simulink model "vehicle_14dof_complete"  (R2025a)
settings: Solver=ode23s  StartTime=0.0  StopTime=10  MaxStep=0.01  RelTol=1e-4  AbsTol=1e-5
model workspace (MAT data in the model file):
  ARB_CONFIG = 2
  MANEUVER_TYPE = 1
  params.vehicle.m = 1905
  params.vehicle.m_s = 1525
  params.vehicle.m_u = 95.5
  params.vehicle.I_xx = 734.04
  params.vehicle.I_yy = 2600
  params.vehicle.I_zz = 2900
  params.vehicle.I_xz = 0
  params.vehicle.I_w = 1
  params.vehicle.a = 1.216
  params.vehicle.b = 1.502
  params.vehicle.L = 2.718
  params.vehicle.w = 1.405
  params.vehicle.t_f = 0.7025
  params.vehicle.t_r = 0.7025
  params.vehicle.hu_cg = 0.5
  params.vehicle.hr_cg = 0.5
  params.vehicle.h_cgM = 0.6629
  params.vehicle.R_w = 0.329
  params.vehicle.k_sf = 75000
  params.vehicle.k_sr = 70000
  params.vehicle.c_sf = 5000
  params.vehicle.c_sr = 4000
  params.vehicle.k_t = 200000
  params.vehicle.L_arb_f = 0.5
  params.vehicle.L_arb_r = 0.5
  params.vehicle.k_arb_f = 12.217304764
  params.vehicle.k_arb_r = 6.98131700798
  params.vehicle.pid_f.Kp = 23.15
  params.vehicle.pid_f.Ki = 10.2
  params.vehicle.pid_f.Kd = 5.4
  params.vehicle.pid_r.Kp = 23.15
  params.vehicle.pid_r.Ki = 10.2
  params.vehicle.pid_r.Kd = 5.4
  params.vehicle.T_aarb_max = 0
  params.vehicle.steering_ratio = 18.5
  params.vehicle.delta_max = 0.698131700798
  params.vehicle.arb_active = 0
  params.tire.mu = 1
  params.tire.mu_r = 0.015
  params.tire.pacejka.fy.a1 = -22.1
  params.tire.pacejka.fy.a2 = 1011
  params.tire.pacejka.fy.a3 = 1078
  params.tire.pacejka.fy.a4 = 1.82
  params.tire.pacejka.fy.a5 = 0.208
  params.tire.pacejka.fy.a6 = 0
  params.tire.pacejka.fy.a7 = -0.354
  params.tire.pacejka.fy.a8 = 0.707
  params.tire.pacejka.fy.C = 1.3
  params.tire.pacejka.fx.a1 = -21.3
  params.tire.pacejka.fx.a2 = 1144
  params.tire.pacejka.fx.a3 = 49.6
  params.tire.pacejka.fx.a4 = 226
  params.tire.pacejka.fx.a5 = 0.069
  params.tire.pacejka.fx.a6 = -0.006
  params.tire.pacejka.fx.a7 = 0.056
  params.tire.pacejka.fx.a8 = 0.486
  params.tire.pacejka.fx.C = 1.65
  params.tire.pacejka.mz.a1 = -2.72
  params.tire.pacejka.mz.a2 = -2.28
  params.tire.pacejka.mz.a3 = -1.86
  params.tire.pacejka.mz.a4 = -2.73
  params.tire.pacejka.mz.a5 = 0.11
  params.tire.pacejka.mz.a6 = -0.07
  params.tire.pacejka.mz.a7 = 0.643
  params.tire.pacejka.mz.a8 = -4.04
  params.tire.pacejka.mz.C = 2.4
  params.sim = struct()
  params.arb_config = 2
  params.arb_name = 'Passive ARB'
  v_initial = 11.1111111111
  x0 = [0; 0; 0.6629; 11.1111111111; 0; 0; 0; 0; 0; 0; 0; 0; -0.0258; -0.0258; -0.0209; -0.0209; 0; 0; 0; 0; 33.7723741979; 33.7723741979; 33.7723741979; 33.7723741979]
settings Model: Creator=Vitor  LastModifiedBy=Vitor
settings DataIOCC: SaveFormat=Array  SaveState=on

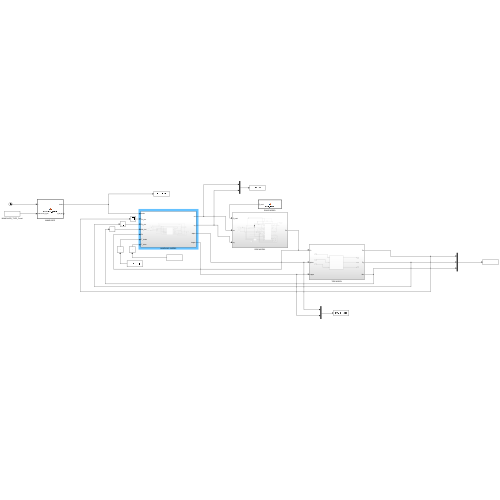
[thumbnail: Simulink's stored preview of the top-level diagram]
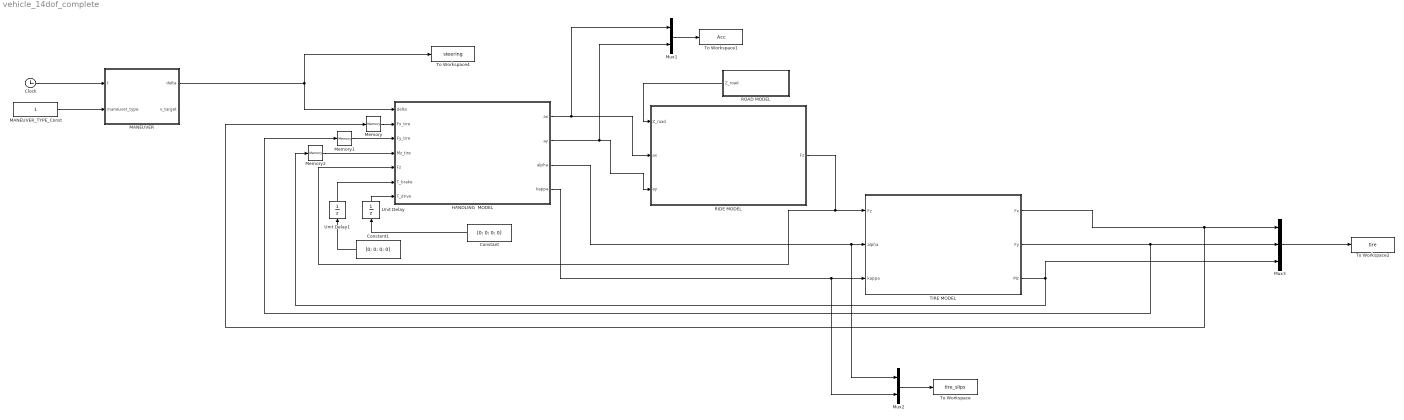
== system vehicle_14dof_complete ==
  Clock : Clock
  Constant : Constant  Value=[0; 0; 0; 0]  SampleTime=0
  Constant1 : Constant  Value=[0; 0; 0; 0]  SampleTime=0
  HANDLING  MODEL : Subsystem
  MANEUVER : MATLAB Function  TreatAsAtomicUnit=on
  MANEUVER_TYPE_Const : Constant  VectorParams1D=off
  Memory : Memory
  Memory1 : Memory
  Memory2 : Memory
  Mux1 : Mux  Inputs=2
  Mux2 : Mux  Inputs=2
  Mux3 : Mux  Inputs=3
  RIDE MODEL : Subsystem
  ROAD MODEL : MATLAB Function  TreatAsAtomicUnit=on
  TIRE MODEL : Subsystem
  To Workspace : ToWorkspace  VariableName=tire_slips  SampleTime=-1
  To Workspace1 : ToWorkspace  VariableName=Acc  SampleTime=-1
  To Workspace2 : ToWorkspace  VariableName=tire  SampleTime=-1
  To Workspace4 : ToWorkspace  VariableName=steering  SampleTime=-1
  Unit Delay : UnitDelay  InitialCondition=[0; 0; 0; 0]  SampleTime=0.01  HasFrameUpgradeWarning=on
  Unit Delay1 : UnitDelay  InitialCondition=[0; 0; 0; 0]  SampleTime=0.01  HasFrameUpgradeWarning=on
  wires:
  MANEUVER_TYPE_Const/1 -> MANEUVER/2(maneuver_type)
  MANEUVER/1(delta) -> To Workspace4/1, HANDLING  MODEL/1(delta)
  ROAD MODEL/1(Z_road) -> RIDE MODEL/1(Z_road)
  Clock/1 -> MANEUVER/1(t)
  TIRE MODEL/1(Fx) -> Memory/1, Mux3/1
  TIRE MODEL/2(Fy) -> Mux3/2, Memory1/1
  TIRE MODEL/3(Mz) -> Memory2/1, Mux3/3
  Mux2/1 -> To Workspace/1
  Mux1/1 -> To Workspace1/1
  Mux3/1 -> To Workspace2/1
  HANDLING  MODEL/1(ax) -> Mux1/1, RIDE MODEL/2(ax)
  HANDLING  MODEL/2(ay) -> Mux1/2, RIDE MODEL/3(ay)
  RIDE MODEL/1(Fz) -> TIRE MODEL/1(Fz), HANDLING  MODEL/5(Fz)
  HANDLING  MODEL/3(alpha) -> Mux2/1, TIRE MODEL/2(alpha)
  HANDLING  MODEL/4(kappa) -> TIRE MODEL/3(kappa), Mux2/2
  Constant/1 -> Unit Delay/1
  Unit Delay/1 -> HANDLING  MODEL/7(T_drive)
  Constant1/1 -> Unit Delay1/1
  Unit Delay1/1 -> HANDLING  MODEL/6(T_brake)
  Memory/1 -> HANDLING  MODEL/2(Fx_tire)
  Memory1/1 -> HANDLING  MODEL/3(Fy_tire)
  Memory2/1 -> HANDLING  MODEL/4(Mz_tire)

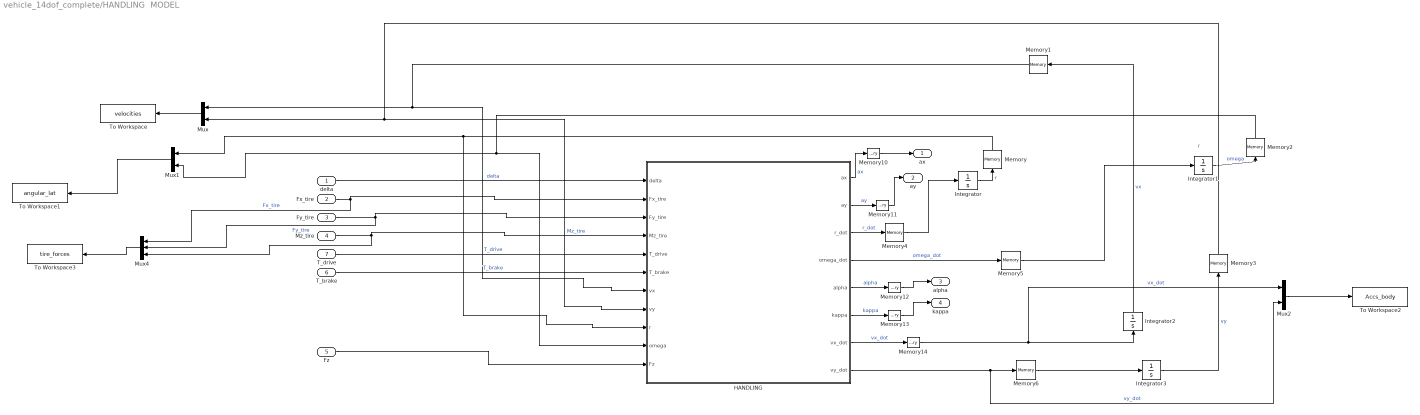
== system vehicle_14dof_complete/HANDLING  MODEL ==
  note: r
  delta : Inport
  Fx_tire : Inport  Port=2
  Fy_tire : Inport  Port=3
  Mz_tire : Inport  Port=4
  Fz : Inport  Port=5
  T_brake : Inport  Port=6
  T_drive : Inport  Port=7
  HANDLING : MATLAB Function  TreatAsAtomicUnit=on
  Integrator : Integrator  InitialCondition=x0(1)
  Integrator1 : Integrator  InitialCondition=x0(2)
  Integrator2 : Integrator  InitialCondition=17.8889
  Integrator3 : Integrator
  Memory{,2..6,10..13} (10 alike) : Memory
  Memory1 : Memory  InitialCondition=11.1111
  Memory14 : Memory  InitialCondition=17.8889
  Mux : Mux  Inputs=2
  Mux1 : Mux  Inputs=2
  Mux2 : Mux  Inputs=2
  Mux4 : Mux  Inputs=3
  To Workspace : ToWorkspace  VariableName=velocities  SampleTime=-1
  To Workspace1 : ToWorkspace  VariableName=angular_lat  SampleTime=-1
  To Workspace2 : ToWorkspace  VariableName=Accs_body  SampleTime=-1
  To Workspace3 : ToWorkspace  VariableName=tire_forces  SampleTime=-1
  ax : Outport
  ay : Outport  Port=2
  alpha : Outport  Port=3
  kappa : Outport  Port=4
  wires:
  delta/1 -> HANDLING/1(delta)  "delta"
  HANDLING/3(r_dot) -> Memory4/1  "r_dot"
  Integrator/1 -> Memory/1  "r"
  HANDLING/4(omega_dot) -> Memory5/1  "omega_dot"
  Integrator1/1 -> Memory2/1  "omega"
  Fx_tire/1 -> Mux4/1, HANDLING/2(Fx_tire)  "Fx_tire"
  Fy_tire/1 -> HANDLING/3(Fy_tire), Mux4/2  "Fy_tire"
  Mz_tire/1 -> HANDLING/4(Mz_tire), Mux4/3  "Mz_tire"
  T_drive/1 -> HANDLING/5(T_drive)  "T_drive"
  T_brake/1 -> HANDLING/6(T_brake)  "T_brake"
  HANDLING/8(vy_dot) -> Mux2/2, Memory6/1  "vy_dot"
  Integrator2/1 -> Memory1/1  "vx"
  Integrator3/1 -> Memory3/1  "vy"
  Mux1/1 -> To Workspace1/1
  Mux2/1 -> To Workspace2/1
  Mux/1 -> To Workspace/1
  Fz/1 -> HANDLING/11(Fz)
  Mux4/1 -> To Workspace3/1
  Memory/1 -> Mux1/1, HANDLING/9(r)
  Memory2/1 -> Mux1/2, HANDLING/10(omega)
  Memory1/1 -> Mux/1, HANDLING/7(vx)
  Memory3/1 -> HANDLING/8(vy), Mux/2
  Memory4/1 -> Integrator/1
  Memory5/1 -> Integrator1/1
  Memory6/1 -> Integrator3/1
  Memory10/1 -> ax/1
  HANDLING/1(ax) -> Memory10/1  "ax"
  HANDLING/2(ay) -> Memory11/1  "ay"
  Memory11/1 -> ay/1
  HANDLING/5(alpha) -> Memory12/1  "alpha"
  HANDLING/6(kappa) -> Memory13/1  "kappa"
  HANDLING/7(vx_dot) -> Memory14/1  "vx_dot"
  Memory12/1 -> alpha/1
  Memory13/1 -> kappa/1
  Memory14/1 -> Mux2/1, Integrator2/1  "vx_dot"

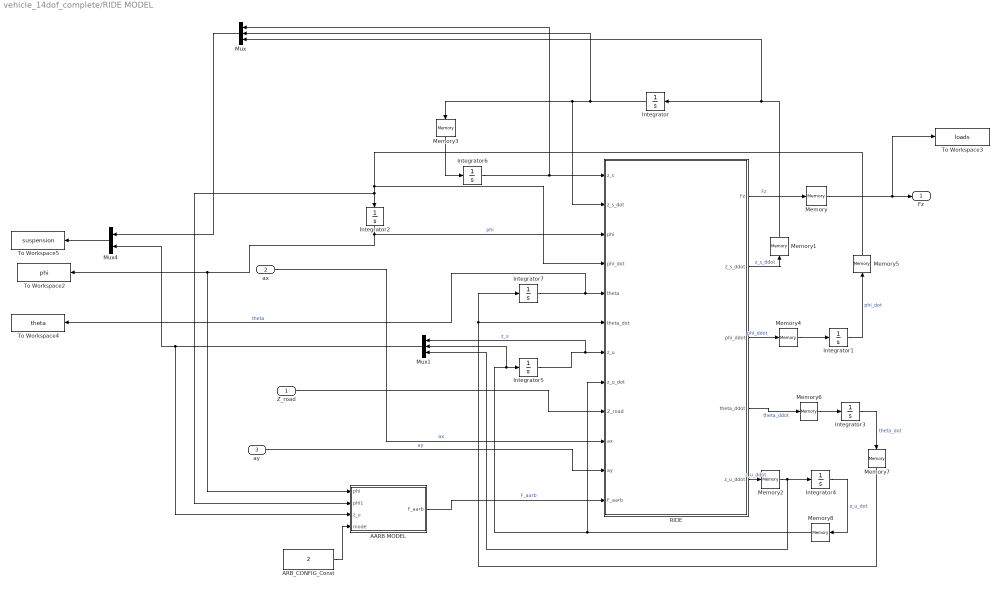
== system vehicle_14dof_complete/RIDE MODEL ==
  Z_road : Inport
  ax : Inport  Port=2
  ay : Inport  Port=3
  AARB MODEL : Subsystem
  ARB_CONFIG_Const : Constant  Value=2
  Integrator : Integrator  InitialCondition=x0(8)
  Integrator1 : Integrator  InitialCondition=x0(9)
  Integrator2 : Integrator  InitialCondition=x0(10)
  Integrator3 : Integrator  InitialCondition=x0(11)
  Integrator4 : Integrator  InitialCondition=x0(12)
  Integrator5 : Integrator  InitialCondition=x0(13)
  Integrator6 : Integrator  InitialCondition=x0(14)
  Integrator7 : Integrator  InitialCondition=x0(15)
  Memory{,1..8} (9 alike) : Memory
  Mux : Mux  Inputs=3
  Mux1 : Mux  Inputs=3
  Mux4 : Mux  Inputs=2
  RIDE : MATLAB Function  TreatAsAtomicUnit=on
  To Workspace2 : ToWorkspace  VariableName=phi  SampleTime=-1
  To Workspace3 : ToWorkspace  VariableName=loads  SampleTime=-1
  To Workspace4 : ToWorkspace  VariableName=theta  SampleTime=-1
  To Workspace5 : ToWorkspace  VariableName=suspension  SampleTime=-1
  Fz : Outport
  wires:
  RIDE/2(z_s_ddot) -> Memory1/1  "z_s_ddot"
  Integrator/1 -> Mux/2, RIDE/2(z_s_dot), Memory3/1
  RIDE/3(phi_ddot) -> Memory4/1  "phi_ddot"
  Integrator1/1 -> Memory5/1  "phi_dot"
  Integrator2/1 -> AARB MODEL/1(phi), To Workspace2/1, RIDE/3(phi)  "phi"
  RIDE/4(theta_ddot) -> Memory6/1  "theta_ddot"
  RIDE/5(z_u_ddot) -> Memory2/1  "z_u_ddot"
  Integrator4/1 -> Memory8/1  "z_u_dot"
  Integrator3/1 -> Memory7/1  "theta_dot"
  Integrator6/1 -> Mux/1, RIDE/1(z_s)
  Integrator7/1 -> To Workspace4/1, RIDE/5(theta)  "theta"
  Z_road/1 -> RIDE/9(Z_road)
  ax/1 -> RIDE/10(ax)  "ax"
  ay/1 -> RIDE/11(ay)  "ay"
  AARB MODEL/1(F_aarb) -> RIDE/12(F_aarb)  "F_aarb"
  Mux/1 -> Mux4/1
  Mux1/1 -> AARB MODEL/3(z_u), Mux4/2
  Integrator5/1 -> Mux1/1, RIDE/7(z_u)  "z_u"
  Mux4/1 -> To Workspace5/1
  Memory1/1 -> Mux/3, Integrator/1
  Memory3/1 -> Integrator6/1
  Memory4/1 -> Integrator1/1
  Memory5/1 -> AARB MODEL/2(phi1), Integrator2/1, RIDE/4(phi_dot)
  Memory6/1 -> Integrator3/1
  Memory7/1 -> RIDE/6(theta_dot), Integrator7/1
  Memory2/1 -> Mux1/3, Integrator4/1
  Memory8/1 -> Mux1/2, Integrator5/1, RIDE/8(z_u_dot)
  RIDE/1(Fz) -> Memory/1  "Fz"
  Memory/1 -> To Workspace3/1, Fz/1
  ARB_CONFIG_Const/1 -> AARB MODEL/4(mode)

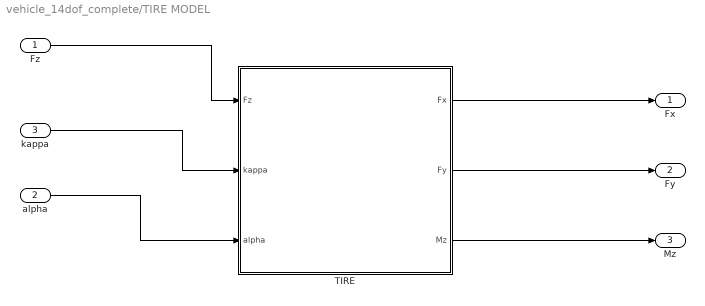
== system vehicle_14dof_complete/TIRE MODEL ==
  Fz : Inport
  alpha : Inport  Port=2
  kappa : Inport  Port=3
  TIRE : MATLAB Function  TreatAsAtomicUnit=on
  Fx : Outport
  Fy : Outport  Port=2
  Mz : Outport  Port=3
  wires:
  kappa/1 -> TIRE/2(kappa)
  TIRE/1(Fx) -> Fx/1
  alpha/1 -> TIRE/3(alpha)
  Fz/1 -> TIRE/1(Fz)
  TIRE/2(Fy) -> Fy/1
  TIRE/3(Mz) -> Mz/1

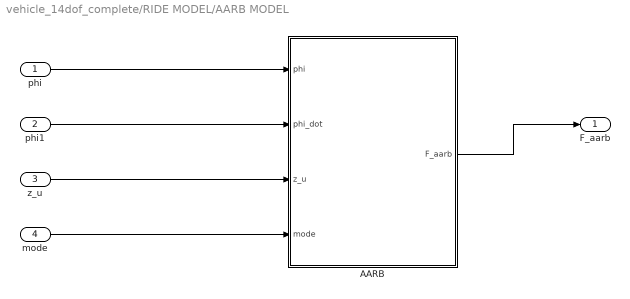
== system vehicle_14dof_complete/RIDE MODEL/AARB MODEL ==
  phi : Inport
  phi1 : Inport  Port=2
  z_u : Inport  Port=3
  mode : Inport  Port=4
  AARB : MATLAB Function  TreatAsAtomicUnit=on
  F_aarb : Outport
  wires:
  phi/1 -> AARB/1(phi)
  AARB/1(F_aarb) -> F_aarb/1
  z_u/1 -> AARB/3(z_u)
  mode/1 -> AARB/4(mode)
  phi1/1 -> AARB/2(phi_dot)

== matlab function vehicle_14dof_complete/RIDE MODEL/AARB MODEL/AARB ==
  data: phi input; phi_dot input; F_aarb output size=[4 1]; z_u input; mode input; params parameter size=[1 3]
function F_aarb = fcn_aarb_controller(phi, phi_dot, z_u, mode, params)
% FCN_AARB_CONTROLLER Calcula forças da barra estabilizadora
%
% Referência: Khalil et al. (2019) - Eqs. 30-33

%% ═══ DECLARAÇÃO EXPLÍCITA DE TAMANHO DE SAÍDA ═══
% Força Simulink a usar tamanho fixo [4×1] para F_aarb
F_aarb = zeros(4, 1);  % ← MOVER PARA PRIMEIRA LINHA EXECUTÁVEL

%% ═══ EXTRAÇÃO DE PARÂMETROS ═══
v = params.vehicle;

% Resto do código...


% Escalares
k_arb_f = v.k_arb_f;
k_arb_r = v.k_arb_r;
L_arb_f = v.L_arb_f;
L_arb_r = v.L_arb_r;
w       = v.w;
T_max   = v.T_aarb_max;

% PID (vetor 1×3)
pid_f = v.pid_f;
pid_r = v.pid_r;

%% ═══ INICIALIZAÇÃO ═══
F_aarb = zeros(4, 1);

%% ═══ SELEÇÃO POR MODO ═══
if mode == 1
    % ════════ NO ARB (Eq. 30) ════════
    F_aarb = zeros(4, 1);
    
elseif mode == 2
    % ════════ PASSIVE ARB (Eq. 31) ════════
    % F = (K_arb * L * Δz) / w
    
    % Dianteira
    delta_z_f = z_u(1) - z_u(2);                    % [m]
    F_f = (k_arb_f * L_arb_f * delta_z_f) / w;      % [N]
    
    F_aarb(1) =  F_f;
    F_aarb(2) = -F_f;
    
    % Traseira
    delta_z_r = z_u(3) - z_u(4);                    % [m]
    F_r = (k_arb_r * L_arb_r * delta_z_r) / w;      % [N]
    
    F_aarb(3) =  F_r;
    F_aarb(4) = -F_r;
    
elseif mode == 3
    % ════════ ACTIVE PID (Eq. 32-33) ════════
    
    Kp_f = pid_f(1);
    Ki_f = pid_f(2);   % Não usado (sem integrador)
    Kd_f = pid_f(3);
    
    % PD simplificado
    T_pid_f = -(Kp_f * phi + Kd_f * phi_dot);
    T_pid_r = T_pid_f;
    
    % Saturação
    T_pid_f = max(min(T_pid_f, T_max), -T_max);
    T_pid_r = max(min(T_pid_r, T_max), -T_max);
    
    % Converter torque em forças
    F_f = T_pid_f / L_arb_f;
    F_r = T_pid_r / L_arb_r;
    
    F_aarb(1) =  F_f;
    F_aarb(2) = -F_f;
    F_aarb(3) =  F_r;
    F_aarb(4) = -F_r;
    
else
    % Modo inválido
    F_aarb = zeros(4, 1);
end

%% ═══ SANEAMENTO FINAL ═══
F_aarb(~isfinite(F_aarb)) = 0;
F_aarb = reshape(F_aarb, 4, 1);

end

== matlab function vehicle_14dof_complete/ROAD MODEL ==
  data: Z_road output double size=[4 1]
function Z_road = road_profile()
%#codegen

Z_road = zeros(4,1);


end

== matlab function vehicle_14dof_complete/RIDE MODEL/RIDE ==
  data: z_s input double size=1; Fz output double size=[4 1]; z_s_dot input double size=1; phi input double size=1; phi_dot input double size=1; theta input double size=1; theta_dot input double size=1; z_u input double size=[4 1]; z_u_dot input double size=[4 1]; Z_road input double size=[4 1]; ax input double size=1; ay input double size=1; F_aarb input double size=[4 1]; z_s_ddot output double size=1; phi_ddot output double size=1; theta_ddot output double size=1; z_u_ddot output double size=[4 1]; params parameter size=1
function [Fz, z_s_ddot, phi_ddot, theta_ddot, z_u_ddot] = ...
    fcn_ride_model(z_s, z_s_dot, phi, phi_dot, theta, theta_dot, ...
    z_u, z_u_dot, Z_road, ax, ay, F_aarb, params)

% coder.extrinsic('struct');   % ← ADICIONAR
% coder.extrinsic('isstruct'); % ← ADICIONAR

%FCN_RIDE_MODEL - Modelo de Ride 7-DOF conforme Khalil et al. (2018)
%
% NOTA: Esta função NÃO usa #codegen para permitir uso de struct params.
%
% ENTRADAS:
%   z_s, z_s_dot       : Deslocamento/velocidade vertical CG [m, m/s]
%   phi, phi_dot       : Ângulo/taxa de roll [rad, rad/s]
%   theta, theta_dot   : Ângulo/taxa de pitch [rad, rad/s]
%   z_u, z_u_dot       : Deslocamentos/velocidades não-suspensas [4x1]
%   Z_road             : Perfil da estrada [4x1] [m]
%   ax, ay             : Acelerações inerciais [m/s²]
%   F_aarb             : Forças AARB [4x1] [N]
%   params             : Struct de parâmetros
%
% SAÍDAS:
%   Fz                 : Forças normais [4x1] [N] (Eq. 26 COMPLETA)
%   z_s_ddot           : Aceleração vertical CG [m/s²] (Eq. 4)
%   phi_ddot           : Aceleração de roll [rad/s²] (Eq. 6)
%   theta_ddot         : Aceleração de pitch [rad/s²] (Eq. 5)
%   z_u_ddot           : Acelerações não-suspensas [4x1] (Eq. 7-10)

%% ═══ INICIALIZAÇÃO ═══
Fz         = zeros(4,1);
z_s_ddot   = 0;
phi_ddot   = 0;
theta_ddot = 0;
z_u_ddot   = zeros(4,1);

%% ═══ PARÂMETROS DO VEÍCULO ═══
v       = params.vehicle;
m_s     = v.m_s;      % Massa suspensa [kg]
m_u     = v.m_u;      % Massa não-suspensa (por roda) [kg]
m_t     = v.m;        % Massa total [kg]
I_xx    = v.I_xx;     % Inércia de roll [kg·m²]
I_yy    = v.I_yy;     % Inércia de pitch [kg·m²]
a       = v.a;        % Distância CG-eixo dianteiro [m]
b       = v.b;        % Distância CG-eixo traseiro [m]
w       = v.w;        % Bitola [m]
hu_cg = v.hu_cg;            % Altura CG ao pitch axis  [m]
hr_cg = v.hr_cg;           % Altura CG ao roll axis [m]
h_cgM = v.h_cgM;              % Altura CG massa suspensa [m]

% Suspensão
K_sf = v.k_sf;  C_sf = v.c_sf;  % Dianteira [N/m, N·s/m]
K_sr = v.k_sr;  C_sr = v.c_sr;  % Traseira [N/m, N·s/m]
K_t  = v.k_t;                    % Rigidez dos pneus [N/m]

% Barra estabilizadora
k_arb_f = v.k_arb_f;  L_arb_f = v.L_arb_f;  % Dianteira
k_arb_r = v.k_arb_r;  L_arb_r = v.L_arb_r;  % Traseira

g = 9.81;  % Gravidade [m/s²]

%% ═══ EQ. 3 - POSIÇÕES E VELOCIDADES NOS CANTOS ═══
% Posição vertical da massa suspensa em cada canto
Z_sfl = z_s - a*theta + 0.5*w*phi;  % Front Left
Z_sfr = z_s - a*theta - 0.5*w*phi;  % Front Right
Z_srl = z_s + b*theta + 0.5*w*phi;  % Rear Left
Z_srr = z_s + b*theta - 0.5*w*phi;  % Rear Right

% Velocidades verticais nos cantos
Z_sfl_dot = z_s_dot - a*theta_dot + 0.5*w*phi_dot;
Z_sfr_dot = z_s_dot - a*theta_dot - 0.5*w*phi_dot;
Z_srl_dot = z_s_dot + b*theta_dot + 0.5*w*phi_dot;
Z_srr_dot = z_s_dot + b*theta_dot - 0.5*w*phi_dot;

%% ═══ EQ. 2 - FORÇAS DE SUSPENSÃO (mola + amortecedor) ═══
F_susp_fl = K_sf*(z_u(1) - Z_sfl) + C_sf*(z_u_dot(1) - Z_sfl_dot);
F_susp_fr = K_sf*(z_u(2) - Z_sfr) + C_sf*(z_u_dot(2) - Z_sfr_dot);
F_susp_rl = K_sr*(z_u(3) - Z_srl) + C_sr*(z_u_dot(3) - Z_srl_dot);
F_susp_rr = K_sr*(z_u(4) - Z_srr) + C_sr*(z_u_dot(4) - Z_srr_dot);

%% ═══ EQ. 4 - ACELERAÇÃO VERTICAL (z_s_ddot) ═══
z_s_ddot = (1/m_s) * ( ...
    - 2*(K_sf + K_sr)*z_s ...
    - 2*(C_sf + C_sr)*z_s_dot ...
    + 2*(a*K_sf - b*K_sr)*theta ...
    + 2*(a*C_sf - b*C_sr)*theta_dot ...
    + K_sf*(z_u(1) + z_u(2)) + C_sf*(z_u_dot(1) + z_u_dot(2)) ...
    + K_sr*(z_u(3) + z_u(4)) + C_sr*(z_u_dot(3) + z_u_dot(4)) );

%% ═══ EQ. 5 - ACELERAÇÃO DE PITCH (theta_ddot) ═══
theta_ddot = (1/I_yy) * ( ...
    - 2*(a^2*K_sf + b^2*K_sr)*theta ...
    - 2*(a^2*C_sf + b^2*C_sr)*theta_dot ...
    + 2*(a*K_sf - b*K_sr)*z_s ...
    + 2*(a*C_sf - b*C_sr)*z_s_dot ...
    - a*K_sf*(z_u(1) + z_u(2)) - a*C_sf*(z_u_dot(1) + z_u_dot(2)) ...
    + b*K_sr*(z_u(3) + z_u(4)) + b*C_sr*(z_u_dot(3) + z_u_dot(4)) ...
    - m_s*hu_cg*ax );

%% ═══ EQ. 6 - ACELERAÇÃO DE ROLL (phi_ddot) ═══
% Momento de roll do ARB (via forças F_aarb)
% F_aarb já inclui o efeito passivo OU ativo, calculado no bloco AARB
M_ARB = -0.5*w*(-F_aarb(1) + F_aarb(2) - F_aarb(3) + F_aarb(4));

phi_ddot = (1/I_xx) * ( ...
    - 0.5*w^2*(K_sf + K_sr)*phi ...
    - 0.5*w^2*(C_sf + C_sr)*phi_dot ...
    + 0.5*w*K_sf*(z_u(1) - z_u(2)) + 0.5*w*C_sf*(z_u_dot(1) - z_u_dot(2)) ...
    + 0.5*w*K_sr*(z_u(3) - z_u(4)) + 0.5*w*C_sr*(z_u_dot(3) - z_u_dot(4)) ...
    + m_s*hr_cg*ay ...
    + M_ARB );  % ✅ Apenas este termo (não duplicar!)


%% ═══ EQ. 7-10 - ACELERAÇÕES NÃO-SUSPENSAS (z_u_ddot) ═══
z_u_ddot(1) = (1/m_u) * ( ...
    -K_sf*(z_u(1) - Z_sfl) - C_sf*(z_u_dot(1) - Z_sfl_dot) ...
    - K_t*(z_u(1) - Z_road(1)) );  % ✅ Removido - F_aarb(1)

z_u_ddot(2) = (1/m_u) * ( ...
    -K_sf*(z_u(2) - Z_sfr) - C_sf*(z_u_dot(2) - Z_sfr_dot) ...
    - K_t*(z_u(2) - Z_road(2)) );  % ✅ Removido - F_aarb(2)

z_u_ddot(3) = (1/m_u) * ( ...
    -K_sr*(z_u(3) - Z_srl) - C_sr*(z_u_dot(3) - Z_srl_dot) ...
    - K_t*(z_u(3) - Z_road(3)) );  % ✅ Removido - F_aarb(3)

z_u_ddot(4) = (1/m_u) * ( ...
    -K_sr*(z_u(4) - Z_srr) - C_sr*(z_u_dot(4) - Z_srr_dot) ...
    - K_t*(z_u(4) - Z_road(4)) );  % ✅ Removido - F_aarb(4)


%% ═══ FORÇAS NORMAIS PARA O PNEU (consistente com RIDE) ═══
% No modelo de ride, o termo do pneu entra como -Kt*(z_u - Z_road) nas Eq. 7-10. [file:2]
delta_z_tire = z_u - Z_road;     % [m]

% Robustez: remove NaN/Inf antes de qualquer operação
delta_z_tire(~isfinite(delta_z_tire)) = 0;

% Força normal (reação vertical do solo no pneu)
Fz = -K_t * delta_z_tire;        % [N]

%% ═══ PROTEÇÃO CONTRA Fz NÃO-POSITIVO/INVÁLIDO ═══
Fz(~isfinite(Fz)) = 100;         % garante não NaN/Inf
Fz = max(Fz, 100);               % garante > 0

% Garantir shape
Fz = reshape(Fz, 4, 1);
end

== matlab function vehicle_14dof_complete/MANEUVER ==
  data: t input; delta output; v_target output; maneuver_type input
function [delta, v_target] = maneuver_profile(t, maneuver_type)
%#codegen
% MANEUVER_PROFILE Gera perfis de esterçamento para Dinâmica Veicular.
% Baseado em normas NHTSA e SAE.
%
% Entradas:
%   t             - Tempo de simulação [s]
%   maneuver_type - Seleção: 1 (Fishhook), 2 (Slowly Increasing Steer)
%
% Saídas:
%   delta         - Ângulo de esterçamento na roda [rad]
%   v_target      - Velocidade longitudinal alvo [m/s]

% ========================================================================
%  DECLARAÇÕES PARA CODE GENERATION
% ========================================================================
% REMOVER TODOS OS coder.extrinsic() QUE NÃO ESTÃO NO TOP-LEVEL

% Inicialização de Variáveis (Garantia para #codegen)
delta_hw_deg = 0.0;     % Ângulo do volante em graus
v_target     = 0.0;     % Velocidade alvo
steering_ratio = 1.0;   % Relação de direção

% ========================================================================
%  PERFIL DA MANOBRA
% ========================================================================
switch maneuver_type
    case 1 % FISHHOOK (NHTSA FMVSS 126)
        % Referência: Khalil et al., 2019 - Figura 16
        % Amplitude: 270° handwheel, Rate: 720°/s
        v_target = 64.4 / 3.6; % 40 mph → m/s
        steering_ratio = 18.5;

        % Timing NHTSA padrão
        t_start = 3.0;           % Início da manobra
        t_ramp1 = 3.375;         % Fim subida (0.375s × 720°/s = 270°)
        t_hold1 = 4.0;           % Fim patamar positivo
        t_ramp2 = 4.75;          % Fim inversão (0.75s × 720°/s = 540° swing)
        t_hold2 = 7.0;           % Fim patamar negativo
        t_ramp3 = 7.375;         % Retorno a zero

        if t < t_start
            delta_hw_deg = 0.0;
        elseif t < t_ramp1
            % Rampa 1: 0 → +270° (720 deg/s)
            delta_hw_deg = 720 * (t - t_start);
        elseif t < t_hold1
            % Dwell 1: Patamar +270°
            delta_hw_deg = 270.0;
        elseif t < t_ramp2
            % Rampa 2: +270° → -270° (720 deg/s)
            delta_hw_deg = 270.0 - 720 * (t - t_hold1);
        elseif t < t_hold2
            % Dwell 2: Patamar -270°
            delta_hw_deg = -270.0;
        elseif t < t_ramp3
            % Rampa 3: -270° → 0° (720 deg/s)
            delta_hw_deg = -270.0 + 720 * (t - t_hold2);
        else
            delta_hw_deg = 0.0;
        end

        % Saturação de segurança (handwheel)
        if delta_hw_deg > 270.0
            delta_hw_deg = 270.0;
        end
        if delta_hw_deg < -270.0
            delta_hw_deg = -270.0;
        end

    case 2 % SLOWLY INCREASING STEER (SAE)
        % Referência: Khalil et al., 2019 - Figura 23
        % Característica: Teste quase-estático para ganho de regime permanente
        v_target = 70 / 3.6;
        steering_ratio = 18.5;

        % Parâmetros temporais
        t_end_ramp = 20.0; % Fim da subida (0 a 270 deg)
        t_end_hold = 22.0; % Fim da sustentação
        t_end_drop = 26.0; % Fim da descida

        if t < 0
            delta_hw_deg = 0.0;
        elseif t <= t_end_ramp
            % Rampa de subida: 270°/20s = 13.5 deg/s
            delta_hw_deg = 13.5 * t;
        elseif t <= t_end_hold
            % Patamar de sustentação (270 deg)
            delta_hw_deg = 270.0;
        elseif t <= t_end_drop
            % Rampa de descida: 270°/4s = 67.5 deg/s
            delta_hw_deg = 270.0 - 67.5 * (t - t_end_hold);
        else
            delta_hw_deg = 0.0;
        end

    otherwise
        % Comportamento padrão seguro (Straight line)
        delta_hw_deg = 0.0;
        v_target = 0.0;
        steering_ratio = 1.0;
end

% ========================================================================
%  PÓS-PROCESSAMENTO CINEMÁTICO
% ========================================================================
% Conversão: Graus Volante → Radianos Roda
delta = (delta_hw_deg / steering_ratio) * (pi / 180);

% Limites Físicos (Saturação Mecânica)
delta_max_physical = 40 * (pi / 180); % ±40° na roda
if abs(delta) > delta_max_physical
    delta = sign(delta) * delta_max_physical;
end

% Garantir tipos corretos (code generation)
delta = double(delta);
v_target = double(v_target);

end

== matlab function vehicle_14dof_complete/TIRE MODEL/TIRE ==
  data: Fz input double size=[4 1]; kappa input double size=[4 1]; Fx output double size=[4 1]; alpha input double size=[4 1]; Fy output double size=[4 1]; Mz output double size=[4 1]; params parameter size=1
function [Fx, Fy, Mz] = fcn_tire_model_pacejka(Fz, kappa, alpha, params)

Fx = zeros(4,1);
Fy = zeros(4,1);
Mz = zeros(4,1);

% ═══ SANITIZAÇÃO MÍNIMA (NECESSÁRIA) ═══
% Garante que Fz não chegue como NaN/Inf/<=0 no assert (especialmente no t=0). [web:12]
Fz = reshape(Fz,4,1);          % garante shape
Fz(~isfinite(Fz)) = 100;       % remove NaN/Inf
Fz = max(Fz, 100);             % impõe mínimo > 0

% Validação mínima
assert(numel(kappa) == 4, '[TIRE] kappa deve ter 4 elementos');
assert(numel(alpha) == 4, '[TIRE] alpha deve ter 4 elementos');
assert(numel(Fz)    == 4, '[TIRE] Fz deve ter 4 elementos');
assert(all(Fz > 0), '[TIRE] Fz deve ser positivo');

% Acesso ao substruct de pneus
t  = params.tire;
mu = t.mu;
fy = t.pacejka.fy;
fx = t.pacejka.fx;
mz = t.pacejka.mz;

% Conversões (conforme notação do artigo)
Fz_kN     = Fz   / 1000;
alpha_deg = alpha * 180/pi;
kappa_pct = kappa * 100;

% Cálculo por roda
for i = 1:4
    Fz_i    = Fz_kN(i);
    alpha_i = alpha_deg(i);
    kappa_i = kappa_pct(i);

    % ===== Eq. 27: Fy =====
    D_y   = fy.a1*Fz_i^2 + fy.a2*Fz_i;
    BCD_y = fy.a3 * sin(2*atan(Fz_i/fy.a4)) * (1 - fy.a5*abs(alpha_i));
    C_y   = fy.C;
    B_y   = BCD_y / (C_y*D_y);
    E_y   = fy.a6*Fz_i^2 + fy.a7*Fz_i + fy.a8;
    arg_y = B_y*alpha_i - E_y*(B_y*alpha_i - atan(B_y*alpha_i));
    Fy(i) = D_y * sin(C_y*atan(arg_y));

    % ===== Eq. 28: Fx =====
    D_x   = fx.a1*Fz_i^2 + fx.a2*Fz_i;
    BCD_x = (fx.a3*Fz_i^2 + fx.a4*Fz_i) * exp(-fx.a5*Fz_i);
    C_x   = fx.C;
    B_x   = BCD_x / (C_x*D_x);
    E_x   = fx.a6*Fz_i^2 + fx.a7*Fz_i + fx.a8;
    arg_x = B_x*kappa_i - E_x*(B_x*kappa_i - atan(B_x*kappa_i));
    Fx(i) = D_x * sin(C_x*atan(arg_x));

    % ===== Eq. 29: Mz =====
    D_m   = mz.a1*Fz_i^2 + mz.a2*Fz_i;
    BCD_m = (mz.a3*Fz_i^2 + mz.a4*Fz_i) * exp(-mz.a5*Fz_i);
    C_m   = mz.C;
    B_m   = BCD_m / (C_m*D_m);
    E_m   = mz.a6*Fz_i^2 + mz.a7*Fz_i + mz.a8;
    arg_m = B_m*alpha_i - E_m*(B_m*alpha_i - atan(B_m*alpha_i));
    Mz(i) = D_m * sin(C_m*atan(arg_m));
end

% Elipse de aderência
for i = 1:4
    F_max   = mu * Fz(i);
    F_total = sqrt(Fx(i)^2 + Fy(i)^2);
    if F_total > F_max
        scale = F_max / F_total;
        Fx(i) = Fx(i)*scale;
        Fy(i) = Fy(i)*scale;
    end
end

% Garantir shapes
Fx = reshape(Fx,4,1);
Fy = reshape(Fy,4,1);
Mz = reshape(Mz,4,1);

end

== matlab function vehicle_14dof_complete/HANDLING  MODEL/HANDLING ==
  data: delta input; Fx_tire input; Fy_tire input; Mz_tire input; T_drive input; T_brake input; ax output double size=1; ay output double size=1; r_dot output double size=1; omega_dot output double size=[4 1]; alpha output double size=[4 1]; kappa output double size=[4 1]; vx_dot output double size=1; vy_dot output double size=1; vx input; vy input; r input; omega input; Fz input; params parameter size=1
function [ax, ay, r_dot, omega_dot, alpha, kappa, vx_dot, vy_dot] = ...
    fcn_handling_model(delta, Fx_tire, Fy_tire, Mz_tire, T_drive, T_brake, ...
    vx, vy, r, omega, Fz, params)
%#codegen
% FCN_HANDLING_MODEL Modelo de dinâmica lateral e longitudinal (14-DOF)
% Referência: Khalil et al., 2019 (Eqs. 11–24)

% Declarações para code generation (mantidas)
coder.extrinsic('struct');
coder.extrinsic('isstruct');

%% 1) Parâmetros do veículo
v    = params.vehicle;
m_t  = v.m;        % Massa total [kg]
I_zz = v.I_zz;     % Inércia de guinada [kg·m²]
w    = v.w;        % Bitola [m]
a    = v.a;        % Distância CG → eixo dianteiro [m]
b    = v.b;        % Distância CG → eixo traseiro [m]
R_w  = v.R_w;      % Raio da roda [m]
I_w  = v.I_w;      % Inércia da roda [kg·m²]

%% 2) Resistência ao rolamento (Tabela 1)
f_r = zeros(4,1);
v_abs = abs(vx);
if v_abs < 1.126
    sigma = 0.0129;
elseif v_abs > 55.555
    sigma = 0.024657;
else
    v_table     = [1.126, 6.944, 13.888, 21.02, 27.777, 34.722, 41.666, 48.423, 55.555];
    sigma_table = [0.0129, 0.0129, 0.01376, 0.014178, 0.015205, 0.016438, 0.0182, 0.021369, 0.024657];
    sigma = interp1(v_table, sigma_table, v_abs, 'linear');
end
for i = 1:4
    f_r(i) = sigma * Fz(i);
end

% %% 3) Cruise control simples (opcional) - DESABILITADO
% T_drive_cc = zeros(4,1);
% v_target = 70/3.6;        % [m/s]
% erro_v   = v_target - vx;
% Kp_cc    = 3000;          % ganho simples
% T_req    = sum(f_r)*R_w + Kp_cc*erro_v;
% if T_req > 0
%     T_drive_cc(3) = T_req/2;   % RWD
%     T_drive_cc(4) = T_req/2;
% end
% T_drive = T_drive + T_drive_cc;

%% 4) Soma das forças longitudinais (Eq. 12)
sum_Fx = 0;
for i = 1:4
    if i <= 2
        sum_Fx = sum_Fx + (Fx_tire(i) - f_r(i))*cos(delta) - Fy_tire(i)*sin(delta);
    else
        sum_Fx = sum_Fx + (Fx_tire(i) - f_r(i));
    end
end
ax = (1/m_t) * sum_Fx;

%% 4.5) Resistência aerodinâmica (Drag + Rolling já aplicado)
% Parâmetros aerodinâmicos (Tabela 1, Khalil 2019)
rho = 1.225;           % Densidade do ar [kg/m³]
Cd = 0.35;             % Coeficiente de arrasto
A_front = 2.5;         % Área frontal [m²]

% Força de arrasto (sempre oposta à velocidade)
F_aero = -0.5 * rho * Cd * A_front * vx * abs(vx);

% Adicionar ao somatório de forças longitudinais
sum_Fx = sum_Fx + F_aero;

ax = (1/m_t) * sum_Fx;

%% 5) Soma das forças laterais (Eq. 14)
sum_Fy = 0;
for i = 1:4
    if i <= 2
        sum_Fy = sum_Fy + (Fx_tire(i) - f_r(i))*sin(delta) + Fy_tire(i)*cos(delta);
    else
        sum_Fy = sum_Fy + Fy_tire(i);
    end
end
ay = (1/m_t) * sum_Fy;

%% 6) Acelerações no corpo (Eqs. 11 e 13)
vx_dot = ax - vy*r;
vy_dot = ay + vx*r;

%% 7) Momento de guinada (Eq. 15 – forma compacta)
% Contribuições principais (longitudinal e lateral transformadas)
Mz_long = 0.5*w * ( (Fx_tire(1)-Fx_tire(2))*cos(delta) + (Fx_tire(3)-Fx_tire(4)) );
Mz_lat  = a*(Fy_tire(1)+Fy_tire(2))*cos(delta) - b*(Fy_tire(3)+Fy_tire(4));
Mz_drag = a*( (Fx_tire(1)-f_r(1))*sin(delta) + (Fx_tire(2)-f_r(2))*sin(delta) );
r_dot   = (1/I_zz) * (Mz_long + Mz_lat + Mz_drag + sum(Mz_tire));

%% 8) Ângulos de deriva (Eqs. 16 e 17) com piso numérico
alpha = zeros(4,1);
vx_min = 0.5;                         % piso para evitar singularidades

if abs(vx) < vx_min
    Vx_eff = sign(vx + 1e-10) * vx_min;  % eps evita sign(0)=0
else
    Vx_eff = vx;
end

% Dianteiras (esterçadas)
alpha(1) = atan2(vy + a*r, Vx_eff) - delta;
alpha(2) = atan2(vy + a*r, Vx_eff) - delta;

% Traseiras
alpha(3) = atan2(vy - b*r, Vx_eff);
alpha(4) = atan2(vy - b*r, Vx_eff);

%% 9) Slip longitudinal κ (Eqs. 18–21) com velocidade ao longo do plano da roda
kappa = zeros(4,1);

% Componentes longitudinais ao plano da roda (frontes incluem delta)
Vwx_f =  vx*cos(delta) + (vy + a*r)*sin(delta);   % aproximação padrão
Vwx_r =  vx;                                      % traseiras (sem esterço)
Vwx    = [Vwx_f; Vwx_f; Vwx_r; Vwx_r];

for i = 1:4
    if abs(Vwx(i)) < vx_min
        Vwx_eff = sign(Vwx(i) + 1e-10) * vx_min;
    else
        Vwx_eff = Vwx(i);
    end
    
    kappa(i) = (omega(i)*R_w - Vwx_eff) / Vwx_eff;
end

%% 10) Aceleração angular das rodas ω̇ (Eq. 24)
omega_dot = zeros(4,1);
for i = 1:4
    % Torque aplicado - Torque de frenagem - Força longitudinal × raio - Resistência × raio
    T_net = T_drive(i) - T_brake(i) - Fx_tire(i)*R_w - f_r(i)*R_w;
    omega_dot(i) = T_net / I_w;
end

%% 11) Saneamento final contra NaN/Inf (robustez)
if ~isfinite(ax),     ax = 0;     end
if ~isfinite(ay),     ay = 0;     end
if ~isfinite(r_dot),  r_dot = 0;  end
if ~isfinite(vx_dot), vx_dot = 0; end
if ~isfinite(vy_dot), vy_dot = 0; end
alpha(~isfinite(alpha))         = 0;
kappa(~isfinite(kappa))         = 0;
omega_dot(~isfinite(omega_dot)) = 0;

%% 12) Garantia de tipos/shapes (codegen)
omega_dot = reshape(double(omega_dot), 4, 1);
alpha     = reshape(double(alpha),     4, 1);
kappa     = reshape(double(kappa),     4, 1);
ax        = double(ax);
ay        = double(ay);
r_dot     = double(r_dot);
vx_dot    = double(vx_dot);
vy_dot    = double(vy_dot);

end
